simulink model "frame_renderer"  (R2014a)
settings: Solver=ode3  StartTime=0.0  StopTime=Inf  RelTol=1e-3
libraries: dspnetwork x1, vrlib x1
settings Model: Creator=Maksim  LastModifiedBy=Maksim
settings DebuggingCC: UnderspecifiedInitializationDetection=Classic  StateNameClashWarn=warning

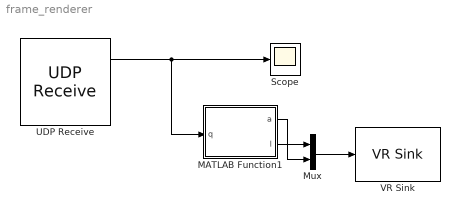
== system frame_renderer ==
  MATLAB Function1 : MATLAB Function  TreatAsAtomicUnit=on
  Mux : Mux  Inputs=2
  Scope : Scope
      settings: YMin=0  YMax=1
  UDP Receive : dspnetwork/UDP Receive  localURL='0.0.0.0'  localPort=18111  remoteURL='0.0.0.0'  remotePort=-1  recvBufferSize=8192  dims=255  signalDatatype=single  isVarSize=off  showBlockingTime=on  blockingTime=inf  sampletime=0.02  blockPlatform=HOST
  VR Sink : vrlib/VR Sink  InstantiateOnLoad=on  SampleTime=-1  ViewEnable=on  RemoteChange=off  RemoteView=off  FieldsWritten=CS.rotation.4.1.1.double  WorldFileName=main.wrl  AutoView=off  VideoDimensions=[]  AllowVariableSize=off
  wires:
  MATLAB Function1/2(l) -> Mux/1
  MATLAB Function1/1(a) -> Mux/2
  Mux/1 -> VR Sink/1
  UDP Receive/1 -> Scope/1, MATLAB Function1/1(q)

== matlab function frame_renderer/MATLAB Function1 ==
  data: a output; q input; l output
function [a, l] = fcn(q)
%#codegen
    % transform the coordinates
    a = 2 * acos(q(1));
    l = q(2:4) / norm(q(2:4));
